simulink model "maglev_LuenbergerObserver"  (R2022b)
settings: Solver=VariableStepAuto  StartTime=0.0  StopTime=10  MaxStep=0.01  RelTol=1e-10
values from neighbouring files (symbols this model uses):
  A = [   0   0  1  0   0 ... (first row only)    [script.m]
  B = [0; 0; 0; 0; -1.5]    [script.m]
  C = [0 0 0 0 1]    [script.m]
  K = [775 48 19 8 -21]    [script.m]
  L = place(A.',C.',lambda_tilde).'    [script.m]
settings Model: Creator=kunde  LastModifiedBy=golovin
settings DebuggingCC: UnconnectedInputMsg=warning  UnconnectedOutputMsg=warning  UnconnectedLineMsg=warning
settings ModelReferenceCC: EnableRefExpFcnMdlSchedulingChecks=on
settings RTWCC: DLArmComputeVersion=19.05

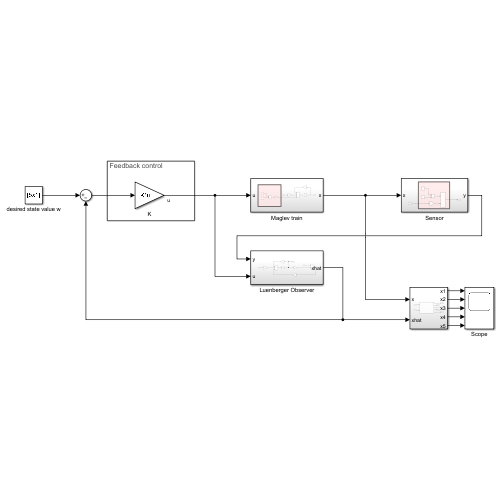
[thumbnail: Simulink's stored preview of the top-level diagram]
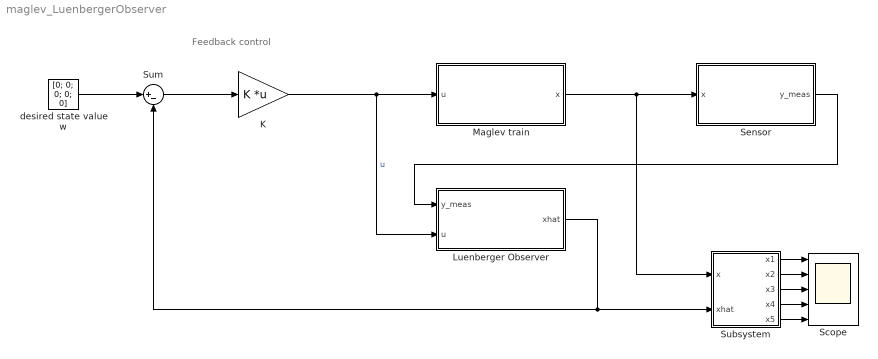
== system maglev_LuenbergerObserver ==
  note: Feedback control
  K : Gain  Gain=K  Multiplication=Matrix(K*u)
  Luenberger Observer : Subsystem
  Maglev train : Subsystem
  Scope : Scope  NumInputPorts=5
  Sensor : Subsystem
  Subsystem : Subsystem
  Sum : Sum  Inputs=|+-
  desired state value w : Constant  Value=[0; 0; 0; 0; 0]
  wires:
  Subsystem/1(x1) -> Scope/1
  Subsystem/2(x2) -> Scope/2
  Subsystem/3(x3) -> Scope/3
  Subsystem/4(x4) -> Scope/4
  Subsystem/5(x5) -> Scope/5
  Luenberger Observer/1(xhat) -> Subsystem/2(xhat), Sum/2
  Maglev train/1(x) -> Subsystem/1(x), Sensor/1(x)
  K/1 -> Luenberger Observer/2(u), Maglev train/1(u)  "u"
  Sum/1 -> K/1
  desired state value w/1 -> Sum/1
  Sensor/1(y_meas) -> Luenberger Observer/1(y_meas)

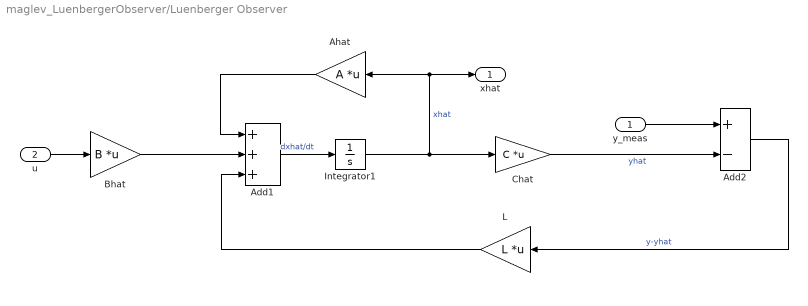
== system maglev_LuenbergerObserver/Luenberger Observer ==
  y_meas : Inport
  u : Inport  Port=2
  Add1 : Sum  Inputs=+++
  Add2 : Sum  Inputs=+-
  Ahat : Gain  Gain=A  Multiplication=Matrix(K*u)
  Bhat : Gain  Gain=B  Multiplication=Matrix(K*u)
  Chat : Gain  Gain=C  Multiplication=Matrix(K*u)
  Integrator1 : Integrator  InitialCondition=[0; 0; 0; 0; 0]
  L : Gain  Gain=L  Multiplication=Matrix(K*u)
  xhat : Outport
  wires:
  Bhat/1 -> Add1/2
  y_meas/1 -> Add2/1
  Integrator1/1 -> Ahat/1, xhat/1, Chat/1  "xhat"
  u/1 -> Bhat/1
  Ahat/1 -> Add1/1
  Add1/1 -> Integrator1/1  "dxhat/dt"
  Chat/1 -> Add2/2  "yhat"
  Add2/1 -> L/1  "y-yhat"
  L/1 -> Add1/3

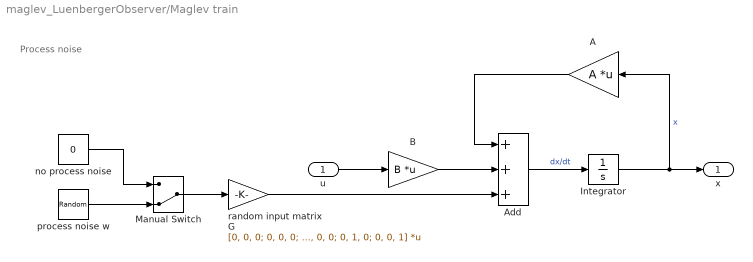
== system maglev_LuenbergerObserver/Maglev train ==
  note: Process noise
  u : Inport
  A : Gain  Gain=A  Multiplication=Matrix(K*u)
  Add : Sum  Inputs=+++
  B : Gain  Gain=B  Multiplication=Matrix(K*u)
  Integrator : Integrator  InitialCondition=[5; 0; 0; 0; 0]
  Manual Switch : ManualSwitch  CurrentSetting=0
  no process noise : Constant  Value=0
  process noise w : RandomNumber  Mean=[0; 0; 0]  Variance=[1; 0.1; 1]/0.01  SampleTime=0.01
  random input matrix G : Gain  Gain=[0, 0, 0; 0, 0, 0; 1, 0, 0; 0, 1, 0; 0, 0, 1]  Multiplication=Matrix(K*u)
  x : Outport
  wires:
  B/1 -> Add/2
  A/1 -> Add/1
  Integrator/1 -> A/1, x/1  "x"
  random input matrix G/1 -> Add/3
  u/1 -> B/1
  Add/1 -> Integrator/1  "dx/dt"
  process noise w/1 -> Manual Switch/2
  Manual Switch/1 -> random input matrix G/1
  no process noise/1 -> Manual Switch/1

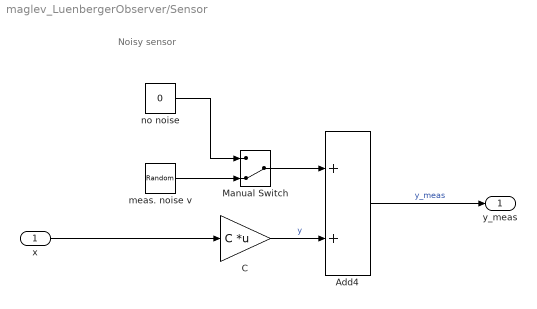
== system maglev_LuenbergerObserver/Sensor ==
  note: Noisy sensor
  x : Inport
  Add4 : Sum
  C : Gain  Gain=C  Multiplication=Matrix(K*u)
  Manual Switch : ManualSwitch  CurrentSetting=0
  meas. noise v : RandomNumber  Variance=1/0.01  SampleTime=0.01
  no noise : Constant  Value=0
  y_meas : Outport
  wires:
  x/1 -> C/1
  C/1 -> Add4/2  "y"
  Add4/1 -> y_meas/1  "y_meas"
  meas. noise v/1 -> Manual Switch/2
  Manual Switch/1 -> Add4/1
  no noise/1 -> Manual Switch/1

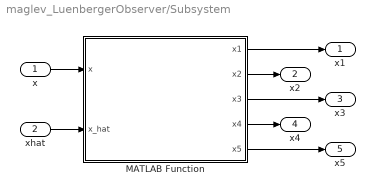
== system maglev_LuenbergerObserver/Subsystem ==
  x : Inport
  xhat : Inport  Port=2
  MATLAB Function : MATLAB Function  TreatAsAtomicUnit=on
  x1 : Outport
  x2 : Outport  Port=2
  x3 : Outport  Port=3
  x4 : Outport  Port=4
  x5 : Outport  Port=5
  wires:
  x/1 -> MATLAB Function/1(x)
  xhat/1 -> MATLAB Function/2(x_hat)
  MATLAB Function/1(x1) -> x1/1
  MATLAB Function/2(x2) -> x2/1
  MATLAB Function/3(x3) -> x3/1
  MATLAB Function/4(x4) -> x4/1
  MATLAB Function/5(x5) -> x5/1

== matlab function maglev_LuenbergerObserver/Subsystem/MATLAB Function ==
  data: x input; x1 output; x_hat input; x2 output; x3 output; x4 output; x5 output
function [x1,x2,x3,x4,x5] = sys_state_comparison(x,x_hat)


x1 = [x(1), x_hat(1)];
x2 = [x(2), x_hat(2)];
x3 = [x(3), x_hat(3)];
x4 = [x(4), x_hat(4)];
x5 = [x(5), x_hat(5)];
